simulink model "G474_curLoop_Decouple"  (R2024a)
settings: Solver=FixedStepAuto  StartTime=0.0  StopTime=10  FixedStep=0.0001  RelTol=1e-3  EnableMultiTasking=on
values from neighbouring files (symbols this model uses):
  currentKi = 1.5    [ACM4010.sldd]
  currentKp = 3.5    [ACM4010.sldd]
  flux = 0.006    [ACM4010.sldd]
  J = 6.0E-6    [ACM4010.sldd]
  Ld = 0.0002    [ACM4010.sldd]
  Lq = 0.0002    [ACM4010.sldd]
  Pn = 5.0    [ACM4010.sldd]
undefined symbols (not defined in the file or in its folder): DiscIntNeverNeededParam, sigbuilder_block
libraries: mcbcontrolslib x5, slpidlib x2, mcbplantlib x1, autolibpmsminterior x1
settings Model: DataDictionary=ACM4010.sldd  Creator=zizhong  LastModifiedBy=zizhong
settings OptimizationCC: DefaultParameterBehavior=Inlined  UseDivisionForNetSlopeComputation=on  GainParamInheritBuiltInType=on  UseFloatMulNetSlope=on  InlineInvariantSignals=on  PassReuseOutputArgsAs=Individual arguments  ZeroExternalMemoryAtStartup=off  ZeroInternalMemoryAtStartup=off  NoFixptDivByZeroProtection=on  EfficientFloat2IntCast=on  LifeSpan=1  MaxStackSize=64  OptimizeBlockOrder=speed  DifferentSizesBufferReuse=on  EfficientTunableParamExpr=on
settings DebuggingCC: ParameterTunabilityLossMsg=error
settings HardwareCC: ProdBitPerPointer=32  ProdBitPerSizeT=32  ProdBitPerPtrDiffT=32  ProdLargestAtomicInteger=Long  ProdLargestAtomicFloat=Double  ProdWordSize=32  ProdLongLongMode=on  ProdHWDeviceType=ARM Compatible->ARM Cortex-M
settings SFSimCC: MATLABDynamicMemAlloc=off  SimTargetLang=C++
settings RTWCC: Description=Embedded Coder  SystemTargetFile=ert.tlc  TemplateMakefile=ert_default_tmf  Toolchain=GNU Tools for ARM Embedded Processors
settings CodeAppCC: ForceParamTrailComments=on  IgnoreCustomStorageClasses=off  OperatorAnnotations=on  SimulinkDataObjDesc=on  SFDataObjDesc=on  CustomSymbolStrGlobalVar=rt$N$M  CustomSymbolStrType=$N$M  CustomSymbolStrFcn=$N$M$F  CustomSymbolStrMacro=$N$M  InsertBlockDesc=on
settings ERTTargetCC: TargetLangStandard=C99 (ISO)  CodeReplacementLibrary=ARM Cortex-M  IncludeMdlTerminateFcn=off  CombineSignalStateStructs=on  SupportComplex=off  SupportNonInlinedSFcns=on  ExtModeTransport=3  ExtModeStaticAlloc=on  ExtModeStaticAllocSize=2048  ExtModeMexFile=ext_xcp  ExtModeIntrfLevel=Level2 - Open  InlinedParameterPlacement=NonHierarchical  ERTCustomFileTemplate=example_file_process.tlc  ERTFilePackagingFormat=CompactWithDataFile

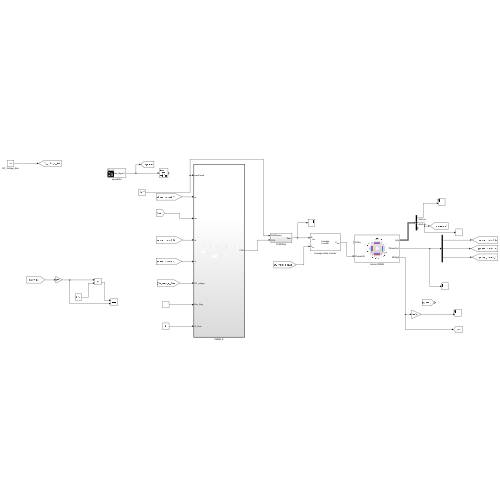
[thumbnail: Simulink's stored preview of the top-level diagram]
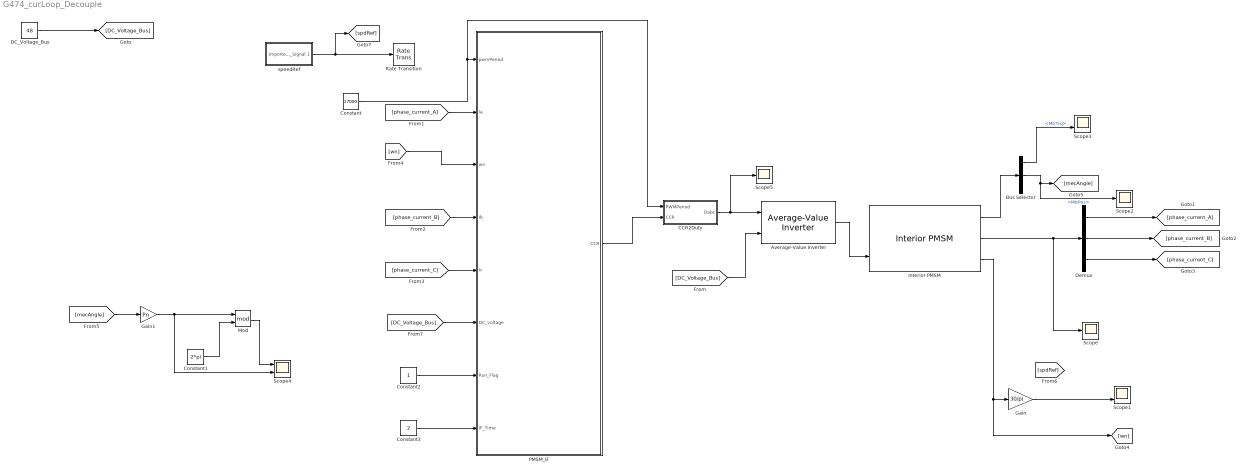
== system G474_curLoop_Decouple ==
  Average-Value Inverter : mcbplantlib/Average-Value Inverter
      settings: LibrarySourceBlock=mcblib/Electrical Systems/Inverters/Average-Value Inverter
  Bus Selector : BusSelector  OutputSignals=MtrTrq,MtrPos,PwrInfo.PwrTrnsfrd
  CCR2Duty : Subsystem
  Constant : Constant  Value=17000
  Constant1 : Constant  Value=2*pi
  Constant2 : Constant
  Constant3 : Constant  Value=2  OutDataTypeStr=single
  DC_Voltage_Bus : Constant  Value=48
  Demux : Demux  Outputs=3
  Gain : Gain  Gain=30/pi
  Gain1 : Gain  Gain=Pn
  Interior PMSM : autolibpmsminterior/Interior PMSM  port_config=Torque  sim_type=Discrete  Ts=0.0001  P=Pn  Rs=Rs  Ldq=[Ld Lq]  KConstText=Permanent flux linkage constant (lambda_pm):  lambda_pm=flux  Ke=159.9771  mechanical=[J,0.924e-4,0]  idq0=[0 0]  theta_init=0  omega_init=0  KConst=flux  lambda_pm_calc=flux  Kt=0.07  RefBlkName='autolibpmsminterior/Interior PMSM'  aMode=5
      settings: LibrarySourceBlock=mcblib/Electrical Systems/Motors/Interior PMSM
  Mod : Math  Operator=mod
  PMSM_IF : Subsystem  TreatAsAtomicUnit=on
      settings: MinAlgLoopOccurrences=on
  Rate Transition : RateTransition
  Scope : Scope
  Scope1 : Scope  NumInputPorts=2
  Scope2 : Scope
  Scope3 : Scope  NumInputPorts=2
  Scope4 : Scope  NumInputPorts=2
  Scope5 : Scope
  speedRef : Subsystem  Tag=STV Subsys  LoadFcn=sigbuilder_block('load');  StartFcn=sigbuilder_block('start');  StopFcn=sigbuilder_block('stop');  ClipboardFcn=sigbuilder_block('clipboard');  mask(Sigbuilder block){tuvar=[0:10]}
      mask help: Simulink:masks:SigbuilderBlock_MD
      mask init:
      | if ~strcmp(get_param(bdroot(gcbh),'SimulationStatus'),'stopped') tuvar = sigbuilder_block('maskInit'); end
      settings: CopyFcn=sigbuilder_block('copy');  DeleteFcn=sigbuilder_block('delete');  ModelCloseFcn=sigbuilder_block('modelClose');  PreSaveFcn=sigbuilder_block('preSave');  PauseFcn=sigbuilder_block('pause');  ContinueFcn=sigbuilder_block('continue');  NameChangeFcn=sigbuilder_block('namechange');  OpenFcn=sigbuilder_block('open',[5.5 36 1269 593 ]);  CloseFcn=sigbuilder_block('close');
      mask Display: plot(0, 0, 100, 100,[2, 2, 32, 32, 2], [68, 8, 8, 68, 68],[32, 2], [38, 38], [32, 19, 2],[53, 60, 44], [32, 17, 17, 2],[16, 16, 31, 31]);txt = getActiveGroup(gcbh);text(2, 100, txt,'verticalAlignment', 'top');
  wires:
  Demux/3 -> [phase_current_C]
  Interior PMSM/2 -> Scope/1, Demux/1
  Average-Value Inverter/1 -> Interior PMSM/2
  CCR2Duty/1(Dabc) -> Scope5/1, Average-Value Inverter/1
  [DC_Voltage_Bus] -> Average-Value Inverter/2
  Bus Selector/1 -> Scope3/2  "<MtrTrq>"
  Gain1/1 -> Scope4/2, Mod/1
  Interior PMSM/3 -> [wn], Gain/1
  Interior PMSM/1 -> Bus Selector/1
  Constant1/1 -> Mod/2
  Demux/1 -> [phase_current_A]
  speedRef/1(Imported_Signal 1) -> Rate Transition/1, [spdRef]
  [mecAngle] -> Gain1/1
  [phase_current_C] -> PMSM_IF/5(Ic)
  Constant/1 -> CCR2Duty/1(PWMPeriod), PMSM_IF/1(pwmPeriod)
  [phase_current_A] -> PMSM_IF/2(Ia)
  Gain/1 -> Scope1/2
  Mod/1 -> Scope4/1
  [phase_current_B] -> PMSM_IF/4(Ib)
  Bus Selector/2 -> Scope2/1, [mecAngle]  "<MtrPos>"
  Demux/2 -> [phase_current_B]
  DC_Voltage_Bus/1 -> [DC_Voltage_Bus]
  [DC_Voltage_Bus] -> PMSM_IF/6(DC_voltage)
  Constant2/1 -> PMSM_IF/7(Run_Flag)
  PMSM_IF/1(CCR) -> CCR2Duty/2(CCR)
  Constant3/1 -> PMSM_IF/8(IF_Time)
  [wn] -> PMSM_IF/3(wn)

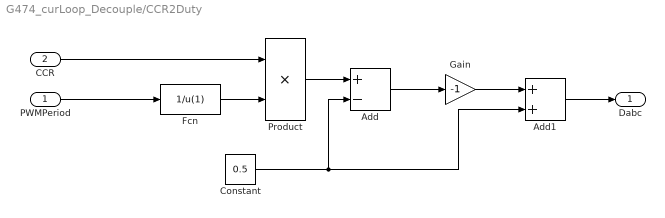
== system G474_curLoop_Decouple/CCR2Duty ==
  PWMPeriod : Inport
  CCR : Inport  Port=2
  Add : Sum  Inputs=+-
  Add1 : Sum
  Constant : Constant  Value=0.5
  Fcn : Fcn  Expr=1/u(1)
  Gain : Gain  Gain=-1
  Product : Product
  Dabc : Outport
  wires:
  PWMPeriod/1 -> Fcn/1
  Fcn/1 -> Product/2
  CCR/1 -> Product/1
  Product/1 -> Add/1
  Constant/1 -> Add1/2, Add/2
  Add/1 -> Gain/1
  Gain/1 -> Add1/1
  Add1/1 -> Dabc/1

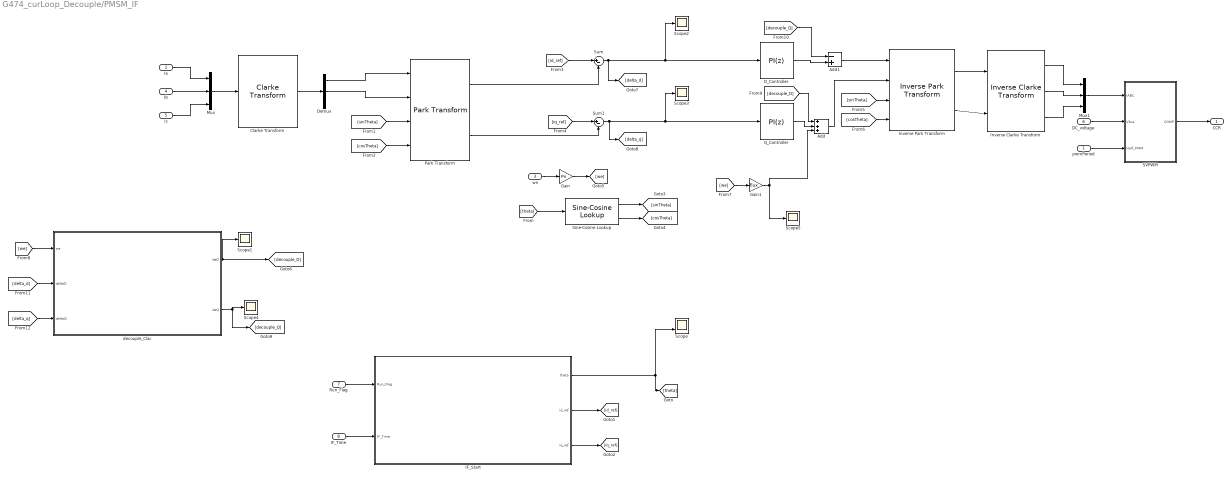
== system G474_curLoop_Decouple/PMSM_IF ==
  pwmPeriod : Inport
  Ia : Inport  Port=2
  wn : Inport  Port=3
  Ib : Inport  Port=4
  Ic : Inport  Port=5
  DC_voltage : Inport  Port=6
  Run_Flag : Inport  Port=7
  IF_Time : Inport  Port=8
  Add : Sum  Inputs=+++
  Add1 : Sum  Inputs=-+
  Clarke Transform : mcbcontrolslib/Clarke Transform  VariantControl=Variant2  PhaseInput=Three inputs  EnPowerInv=off
      settings: LibrarySourceBlock=mcbhdllib/Controls/Math Transforms/Clarke Transform
  D_Controller : slpidlib/PID Controller  Controller=PI  Form=Parallel  TimeDomain=Discrete-time  UseExternalTs=off  SampleTime=-1  IntegratorMethod=Forward Euler  FilterMethod=Forward Euler  ControllerParametersSource=internal  P=currentKp  I=currentKi  UseKiTs=off  D=0  UseExternalDerivativeSource=off  N=100  UseFilter=on  TunerSelectOption=Transfer Function Based (PID Tuner App)  InitialConditionSource=internal  InitialConditionForIntegrator=0  InitialConditionForFilter=0  DifferentiatorICPrevScaledInput=0  ExternalReset=none  TrackingMode=off  Kt=1  LimitOutput=on  SatLimitsSource=internal  UpperSaturationLimit=12  LowerSaturationLimit=-12  LinearizeAsGain=on  AntiWindupMode=clamping  Kb=1  LimitIntegrator=off  UpperIntegratorSaturationLimit=inf  LowerIntegratorSaturationLimit=-inf  PGainOutDataTypeStr=single  PProdOutDataTypeStr=single  POutMin=[]  POutMax=[]  IGainOutDataTypeStr=int16  IProdOutDataTypeStr=int16  IOutMin=[]  IOutMax=[]  DOutMin=[]  DOutMax=[]  NOutMin=[]  NOutMax=[]  SumOutDataTypeStr=single  SumOutMin=[]  SumOutMax=[]  SaturationOutDataTypeStr=single  SaturationOutMin=[]  SaturationOutMax=[]  PParamMin=[]  PParamMax=[]  IParamMin=[]  IParamMax=[]  DParamMin=[]  DParamMax=[]  NParamMin=[]  NParamMax=[]  KbParamMin=[]  KbParamMax=[]  KtParamMin=[]  KtParamMax=[]  KbOutMin=[]  KbOutMax=[]  KtOutMin=[]  KtOutMax=[]  IntegratorOutMin=[]  IntegratorOutMax=[]  FilterOutMin=[]  FilterOutMax=[]  SumI1OutMin=[]  SumI1OutMax=[]  SumI2OutMin=[]  SumI2OutMax=[]  SumI3OutMin=[]  SumI3OutMax=[]  SumI4OutMin=[]  SumI4OutMax=[]  SumDOutMin=[]  SumDOutMax=[]  DifferentiatorOutMin=[]  DifferentiatorOutMax=[]  FilterDiffOutCoefMin=[]  FilterDiffOutCoefMax=[]  ReciprocalOutMin=[]  ReciprocalOutMax=[]  SumDenOutMin=[]  SumDenOutMax=[]  SumNumOutMin=[]  SumNumOutMax=[]  DivideOutMin=[]  DivideOutMax=[]  UdiffTsProdOutMin=[]  UdiffTsProdOutMax=[]  NTsProdOutMin=[]  NTsProdOutMax=[]  UintegralTsProdOutMin=[]  UintegralTsProdOutMax=[]  UngainTsProdOutMin=[]  UngainTsProdOutMax=[]  ClampingZeroOutDataTypeStr=Inherit: Inherit via back propagation  ClampingZeroOutMin=[]  ClampingZeroOutMax=[]  FilterDenConstantOutDataTypeStr=Inherit: Inherit via back propagation  FilterDenConstantOutMin=[]  FilterDenConstantOutMax=[]  PCopyOutDataTypeStr=Inherit: Inherit via back propagation  PCopyOutMin=[]  PCopyOutMax=[]  NCopyOutDataTypeStr=Inherit: Inherit via back propagation  NCopyOutMin=[]  NCopyOutMax=[]  IntegratorContinuousStateAttributes=''  IntegratorStateMustResolveToSignalObject=off  IntegratorRTWStateStorageClass=Auto  FilterContinuousStateAttributes=''  FilterStateMustResolveToSignalObject=off  FilterRTWStateStorageClass=Auto  ParallelPVariant=InternalParameters  IdealPVariant=Disabled  IVariant=InternalParameters  DVariant=Disabled  IntegratorVariant=Discrete  SatVariant=Enabled  AWVariant=DiscClampingParallel  PCopyVariant=Disabled  TRVariant=Disabled  FdbkBlocksVariant=Forward  IdealPFdbkVariant=Disabled  SatFdbkVariant=Disabled  DerivativeFilterVariant=Disabled  NVariant=Disabled  NCopyVariant=Disabled_SignalSpec  FilterICVariant=Disabled  IntegratorICVariant=InternalICs  ExternalResetVariant=Disabled  TRSumVariant=Passthrough  SumFdbkVariant=Disabled  SumVariant=Sum_PI  TsampFilterVariant=InternalTs  TsampNgainVariant=Passthrough  TsampIntegralVariant=Disabled_SignalSpec  ExternalSaturationOutDataTypeStr=Inherit: Same as second input  DerivativeSourceVariant=Disabled
  Demux : Demux  Outputs=3
  Gain : Gain  Gain=Pn
  Gain1 : Gain  Gain=flux
  IF_Start : Subsystem  TreatAsAtomicUnit=on
      settings: MinAlgLoopOccurrences=on
  Inverse Clarke Transform : mcbcontrolslib/Inverse Clarke Transform  PhaseInput=Two inputs  EnPowerInv=off
      settings: LibrarySourceBlock=mcbhdllib/Controls/Math Transforms/Inverse Clarke Transform
  Inverse Park Transform : mcbcontrolslib/Inverse Park Transform  PhaseInput=Two inputs  AxisAlignment=D-axis  ThetaInput=Sine and Cosine electrical position  AngleInput=Per-unit  N_points=1024
      settings: LibrarySourceBlock=mcbhdllib/Controls/Math Transforms/Inverse Park Transform
  Mux : Mux  Inputs=3
  Mux1 : Mux  Inputs=3
  Park Transform : mcbcontrolslib/Park Transform  PhaseInput=Two inputs  AxisAlignment=D-axis  ThetaInput=Sine and Cosine electrical position  AngleInput=Per-unit  N_points=1024
      settings: LibrarySourceBlock=mcbhdllib/Controls/Math Transforms/Park Transform
  Q_Controller : slpidlib/PID Controller  Controller=PI  Form=Parallel  TimeDomain=Discrete-time  UseExternalTs=off  SampleTime=-1  IntegratorMethod=Forward Euler  FilterMethod=Forward Euler  ControllerParametersSource=internal  P=currentKp  I=currentKi  UseKiTs=off  D=0  UseExternalDerivativeSource=off  N=100  UseFilter=on  TunerSelectOption=Transfer Function Based (PID Tuner App)  InitialConditionSource=internal  InitialConditionForIntegrator=0  InitialConditionForFilter=0  DifferentiatorICPrevScaledInput=0  ExternalReset=none  TrackingMode=off  Kt=1  LimitOutput=on  SatLimitsSource=internal  UpperSaturationLimit=12  LowerSaturationLimit=-12  LinearizeAsGain=on  AntiWindupMode=clamping  Kb=1  LimitIntegrator=off  UpperIntegratorSaturationLimit=inf  LowerIntegratorSaturationLimit=-inf  PGainOutDataTypeStr=single  PProdOutDataTypeStr=single  POutMin=[]  POutMax=[]  IGainOutDataTypeStr=int16  IProdOutDataTypeStr=int16  IOutMin=[]  IOutMax=[]  DOutMin=[]  DOutMax=[]  NOutMin=[]  NOutMax=[]  SumOutDataTypeStr=single  SumOutMin=[]  SumOutMax=[]  SaturationOutDataTypeStr=single  SaturationOutMin=[]  SaturationOutMax=[]  PParamMin=[]  PParamMax=[]  IParamMin=[]  IParamMax=[]  DParamMin=[]  DParamMax=[]  NParamMin=[]  NParamMax=[]  KbParamMin=[]  KbParamMax=[]  KtParamMin=[]  KtParamMax=[]  KbOutMin=[]  KbOutMax=[]  KtOutMin=[]  KtOutMax=[]  IntegratorOutMin=[]  IntegratorOutMax=[]  FilterOutMin=[]  FilterOutMax=[]  SumI1OutMin=[]  SumI1OutMax=[]  SumI2OutMin=[]  SumI2OutMax=[]  SumI3OutMin=[]  SumI3OutMax=[]  SumI4OutMin=[]  SumI4OutMax=[]  SumDOutMin=[]  SumDOutMax=[]  DifferentiatorOutMin=[]  DifferentiatorOutMax=[]  FilterDiffOutCoefMin=[]  FilterDiffOutCoefMax=[]  ReciprocalOutMin=[]  ReciprocalOutMax=[]  SumDenOutMin=[]  SumDenOutMax=[]  SumNumOutMin=[]  SumNumOutMax=[]  DivideOutMin=[]  DivideOutMax=[]  UdiffTsProdOutMin=[]  UdiffTsProdOutMax=[]  NTsProdOutMin=[]  NTsProdOutMax=[]  UintegralTsProdOutMin=[]  UintegralTsProdOutMax=[]  UngainTsProdOutMin=[]  UngainTsProdOutMax=[]  ClampingZeroOutDataTypeStr=Inherit: Inherit via back propagation  ClampingZeroOutMin=[]  ClampingZeroOutMax=[]  FilterDenConstantOutDataTypeStr=Inherit: Inherit via back propagation  FilterDenConstantOutMin=[]  FilterDenConstantOutMax=[]  PCopyOutDataTypeStr=Inherit: Inherit via back propagation  PCopyOutMin=[]  PCopyOutMax=[]  NCopyOutDataTypeStr=Inherit: Inherit via back propagation  NCopyOutMin=[]  NCopyOutMax=[]  IntegratorContinuousStateAttributes=''  IntegratorStateMustResolveToSignalObject=off  IntegratorRTWStateStorageClass=Auto  FilterContinuousStateAttributes=''  FilterStateMustResolveToSignalObject=off  FilterRTWStateStorageClass=Auto  ParallelPVariant=InternalParameters  IdealPVariant=Disabled  IVariant=InternalParameters  DVariant=Disabled  IntegratorVariant=Discrete  SatVariant=Enabled  AWVariant=DiscClampingParallel  PCopyVariant=Disabled  TRVariant=Disabled  FdbkBlocksVariant=Forward  IdealPFdbkVariant=Disabled  SatFdbkVariant=Disabled  DerivativeFilterVariant=Disabled  NVariant=Disabled  NCopyVariant=Disabled_SignalSpec  FilterICVariant=Disabled  IntegratorICVariant=InternalICs  ExternalResetVariant=Disabled  TRSumVariant=Passthrough  SumFdbkVariant=Disabled  SumVariant=Sum_PI  TsampFilterVariant=InternalTs  TsampNgainVariant=Passthrough  TsampIntegralVariant=Disabled_SignalSpec  ExternalSaturationOutDataTypeStr=Inherit: Same as second input  DerivativeSourceVariant=Disabled
  SVPWM : Subsystem  TreatAsAtomicUnit=on
      settings: MinAlgLoopOccurrences=on
  Scope : Scope  NumInputPorts=2
  Scope{1..5} (5 alike) : Scope
  Sine-Cosine Lookup : mcbcontrolslib/Sine-Cosine Lookup  AngleInput=Radians  N_points=1024  DatatypeInput=Inherit from input  Datatype=single
      settings: LibrarySourceBlock=mcblib/Controls/Math Transforms/Sine-Cosine Lookup
  Sum : Sum  Inputs=|+-
  Sum1 : Sum  Inputs=|+-
  decouple_Clac : Subsystem
  CCR : Outport
  wires:
  [theta] -> Sine-Cosine Lookup/1
  Mux/1 -> Clarke Transform/1
  Ia/1 -> Mux/1
  Ib/1 -> Mux/2
  Ic/1 -> Mux/3
  Sine-Cosine Lookup/1 -> [sinTheta]
  Sine-Cosine Lookup/2 -> [cosTheta]
  [sinTheta] -> Park Transform/3
  [cosTheta] -> Park Transform/4
  Clarke Transform/1 -> Demux/1
  Demux/2 -> Park Transform/2
  Demux/1 -> Park Transform/1
  Park Transform/1 -> Sum/2
  Park Transform/2 -> Sum1/2
  [id_ref] -> Sum/1
  [iq_ref] -> Sum1/1
  [sinTheta] -> Inverse Park Transform/3
  [cosTheta] -> Inverse Park Transform/4
  Inverse Park Transform/1 -> Inverse Clarke Transform/1
  Inverse Park Transform/2 -> Inverse Clarke Transform/2
  Inverse Clarke Transform/1 -> Mux1/1
  Inverse Clarke Transform/2 -> Mux1/2
  Inverse Clarke Transform/3 -> Mux1/3
  Mux1/1 -> SVPWM/1(IABC)
  DC_voltage/1 -> SVPWM/2(Vbus)
  pwmPeriod/1 -> SVPWM/3(Half_PWM)
  SVPWM/1(COMP) -> CCR/1
  IF_Start/1(theta) -> Scope/2, [theta]
  Run_Flag/1 -> IF_Start/1(Run_Flag)
  IF_Time/1 -> IF_Start/2(IF_Time)
  IF_Start/2(id_ref) -> [id_ref]
  IF_Start/3(iq_ref) -> [iq_ref]
  Add/1 -> Inverse Park Transform/2
  Add1/1 -> Inverse Park Transform/1
  D_Controller/1 -> Add1/2
  wn/1 -> Gain/1
  Gain/1 -> [we]
  [we] -> Gain1/1
  Q_Controller/1 -> Add/2
  [decouple_D] -> Add/1
  [decouple_Q] -> Add1/1
  Gain1/1 -> Add/3, Scope5/1
  decouple_Clac/2(deQ) -> [decouple_Q], Scope4/1
  decouple_Clac/1(deD) -> [decouple_D], Scope1/1
  [we] -> decouple_Clac/1(we)
  [delta_d] -> decouple_Clac/2(deltaD)
  [delta_q] -> decouple_Clac/3(deltaQ)
  Sum1/1 -> [delta_q], Q_Controller/1, Scope3/1
  Sum/1 -> [delta_d], D_Controller/1, Scope2/1

== system G474_curLoop_Decouple/speedRef ==
  Demux : Demux  Tag=STV Demux  Outputs=1
      settings: DisplayOption=none
  FromWs : FromWorkspace  Tag=STV FromWs  VariableName=tuvar
      SigBuilderData=|
      | common.afterFinalStr = 'Extrapolate'
      | common.sampleTime = 0
      | dataSet.timeRange = [0 10]
      | dataSet.name = 'Sheet1'
      | sbobj.Groups.Name = 'Sheet1'
      | sbobj.Groups.Signals.Name = 'Imported_Signal 1'
      | sbobj.Groups.Signals.XData = [0 1 2 3 4 5 5.96 7 8 9 10]
      | sbobj.Groups.Signals.YData = [3580 3680 3785 3660 3855 3595 3670 3535 2755 3650 3760]
  Imported_Signal 1 : Outport  Tag=STV Outport
  wires:
  Demux/1 -> Imported_Signal 1/1
  FromWs/1 -> Demux/1

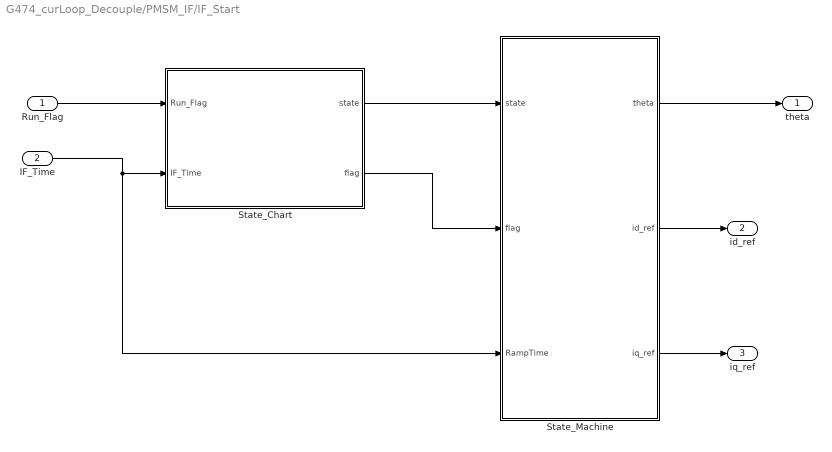
== system G474_curLoop_Decouple/PMSM_IF/IF_Start ==
  Run_Flag : Inport
  IF_Time : Inport  Port=2
  State_Chart : Stateflow chart
      settings: MinAlgLoopOccurrences=on
  State_Machine : Subsystem  TreatAsAtomicUnit=on
      settings: MinAlgLoopOccurrences=on
  theta : Outport
  id_ref : Outport  Port=2
  iq_ref : Outport  Port=3
  wires:
  State_Machine/3(iq_ref) -> iq_ref/1
  State_Chart/2(flag) -> State_Machine/2(flag)
  IF_Time/1 -> State_Machine/3(RampTime), State_Chart/2(IF_Time)
  State_Chart/1(state) -> State_Machine/1(state)
  State_Machine/1(theta) -> theta/1
  State_Machine/2(id_ref) -> id_ref/1
  Run_Flag/1 -> State_Chart/1(Run_Flag)

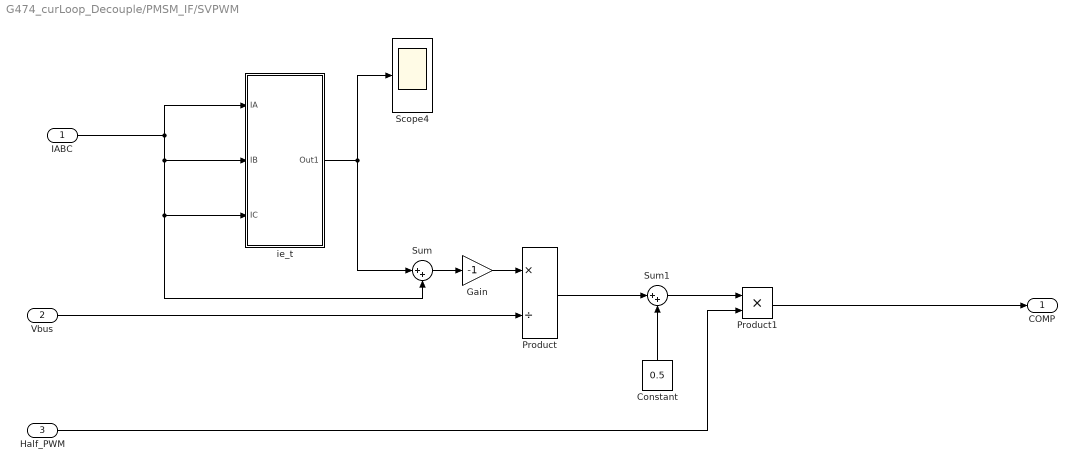
== system G474_curLoop_Decouple/PMSM_IF/SVPWM ==
  IABC : Inport
  Vbus : Inport  Port=2
  Half_PWM : Inport  Port=3
  Constant : Constant  Value=0.5
  Gain : Gain  Gain=-1
  Product : Product  Inputs=*/
  Product1 : Product
  Scope4 : Scope
  Sum : Sum  Inputs=|++
  Sum1 : Sum  Inputs=|++
  ie_t : Subsystem
  COMP : Outport
  wires:
  IABC/1 -> ie_t/3(IC), Sum/2, ie_t/2(IB), ie_t/1(IA)
  Half_PWM/1 -> Product1/2
  Gain/1 -> Product/1
  ie_t/1(Out1) -> Sum/1, Scope4/1
  Sum/1 -> Gain/1
  Sum1/1 -> Product1/1
  Constant/1 -> Sum1/2
  Product/1 -> Sum1/1
  Vbus/1 -> Product/2
  Product1/1 -> COMP/1

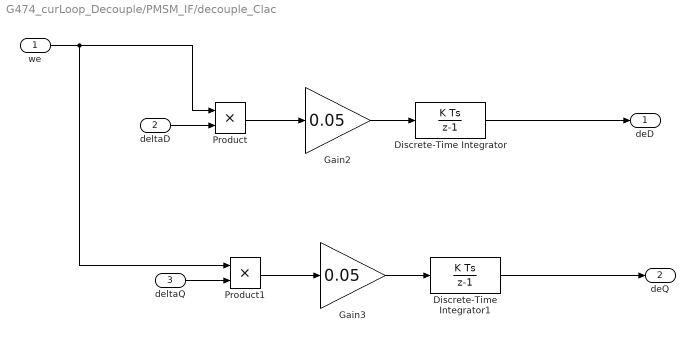
== system G474_curLoop_Decouple/PMSM_IF/decouple_Clac ==
  we : Inport
  deltaD : Inport  Port=2
  deltaQ : Inport  Port=3
  Discrete-Time Integrator : DiscreteIntegrator  SampleTime=-1  LimitOutput=on  UpperSaturationLimit=8  LowerSaturationLimit=-8  ICPrevOutput=DiscIntNeverNeededParam  ICPrevScaledInput=DiscIntNeverNeededParam
  Discrete-Time Integrator1 : DiscreteIntegrator  SampleTime=-1  LimitOutput=on  UpperSaturationLimit=8  LowerSaturationLimit=-8  ICPrevOutput=DiscIntNeverNeededParam  ICPrevScaledInput=DiscIntNeverNeededParam
  Gain2 : Gain  Gain=0.05
  Gain3 : Gain  Gain=0.05
  Product : Product
  Product1 : Product
  deD : Outport
  deQ : Outport  Port=2
  wires:
  Gain2/1 -> Discrete-Time Integrator/1
  Product/1 -> Gain2/1
  we/1 -> Product1/1, Product/1
  Product1/1 -> Gain3/1
  Gain3/1 -> Discrete-Time Integrator1/1
  Discrete-Time Integrator/1 -> deD/1
  deltaQ/1 -> Product1/2
  deltaD/1 -> Product/2
  Discrete-Time Integrator1/1 -> deQ/1

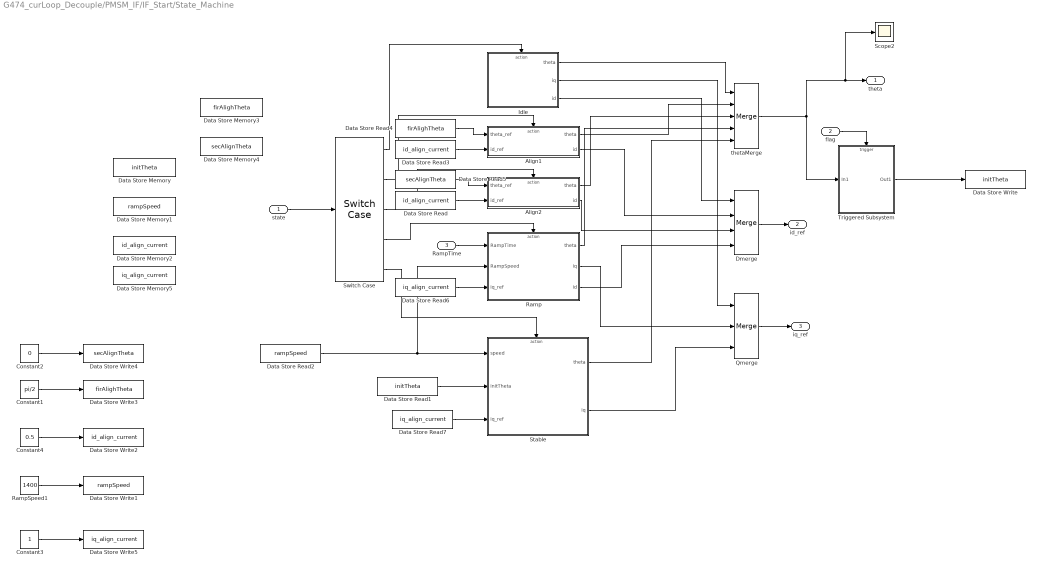
== system G474_curLoop_Decouple/PMSM_IF/IF_Start/State_Machine ==
  state : Inport
  flag : Inport  Port=2
  RampTime : Inport  Port=3
  Align1 : Subsystem  TreatAsAtomicUnit=on
  Align2 : Subsystem  TreatAsAtomicUnit=on
  Constant1 : Constant  Value=pi/2  OutDataTypeStr=single
  Constant2 : Constant  Value=0  OutDataTypeStr=single
  Constant3 : Constant  OutDataTypeStr=single
  Constant4 : Constant  Value=0.5  OutDataTypeStr=single
  Data Store Memory : DataStoreMemory  DataStoreName=initTheta  WriteAfterWriteMsg=warning  ShowAdditionalParam=off
  Data Store Memory1 : DataStoreMemory  DataStoreName=rampSpeed  WriteAfterWriteMsg=warning  ShowAdditionalParam=off
  Data Store Memory2 : DataStoreMemory  DataStoreName=id_align_current  WriteAfterWriteMsg=warning  ShowAdditionalParam=off
  Data Store Memory3 : DataStoreMemory  DataStoreName=firAlighTheta  WriteAfterWriteMsg=warning  ShowAdditionalParam=off
  Data Store Memory4 : DataStoreMemory  DataStoreName=secAlignTheta  WriteAfterWriteMsg=warning  ShowAdditionalParam=off
  Data Store Memory5 : DataStoreMemory  DataStoreName=iq_align_current  WriteAfterWriteMsg=warning  ShowAdditionalParam=off
  Data Store Read : DataStoreRead  DataStoreName=id_align_current  IndexOptions=Index vector (dialog)  Indices=1  OutputSizes=1
  Data Store Read1 : DataStoreRead  DataStoreName=initTheta  IndexOptions=Index vector (dialog)  Indices=1  OutputSizes=1
  Data Store Read2 : DataStoreRead  DataStoreName=rampSpeed  IndexOptions=Index vector (dialog)  Indices=1  OutputSizes=1
  Data Store Read3 : DataStoreRead  DataStoreName=id_align_current  IndexOptions=Index vector (dialog)  Indices=1  OutputSizes=1
  Data Store Read4 : DataStoreRead  DataStoreName=firAlighTheta  IndexOptions=Index vector (dialog)  Indices=1  OutputSizes=1
  Data Store Read5 : DataStoreRead  DataStoreName=secAlignTheta  IndexOptions=Index vector (dialog)  Indices=1  OutputSizes=1
  Data Store Read6 : DataStoreRead  DataStoreName=iq_align_current  IndexOptions=Index vector (dialog)  Indices=1  OutputSizes=1
  Data Store Read7 : DataStoreRead  DataStoreName=iq_align_current  IndexOptions=Index vector (dialog)  Indices=1  OutputSizes=1
  Data Store Write : DataStoreWrite  DataStoreName=initTheta  IndexOptions=Index vector (dialog)  Indices=1  OutputSizes=1
  Data Store Write1 : DataStoreWrite  DataStoreName=rampSpeed  IndexOptions=Index vector (dialog)  Indices=1  OutputSizes=1
  Data Store Write2 : DataStoreWrite  DataStoreName=id_align_current  IndexOptions=Index vector (dialog)  Indices=1  OutputSizes=1
  Data Store Write3 : DataStoreWrite  DataStoreName=firAlighTheta  IndexOptions=Index vector (dialog)  Indices=1  OutputSizes=1
  Data Store Write4 : DataStoreWrite  DataStoreName=secAlignTheta  IndexOptions=Index vector (dialog)  Indices=1  OutputSizes=1
  Data Store Write5 : DataStoreWrite  DataStoreName=iq_align_current  IndexOptions=Index vector (dialog)  Indices=1  OutputSizes=1
  Dmerge : Merge  Inputs=4
  Idle : Subsystem  TreatAsAtomicUnit=on
  Qmerge : Merge  Inputs=3
  Ramp : Subsystem  TreatAsAtomicUnit=on
  RampSpeed1 : Constant  Value=1400  OutDataTypeStr=single
  Scope2 : Scope
  Stable : Subsystem  TreatAsAtomicUnit=on
  Switch Case : SwitchCase  CaseConditions={0, 1, 2, 3, 4}  ShowDefaultCase=off
  Triggered Subsystem : Subsystem  TreatAsAtomicUnit=on
  thetaMerge : Merge  Inputs=5
  theta : Outport
  id_ref : Outport  Port=2
  iq_ref : Outport  Port=3
  wires:
  Align1/2(id) -> Dmerge/2
  Data Store Read4/1 -> Align1/1(theta_ref)
  Switch Case/5 -> Stable/Action
  Switch Case/1 -> Idle/Action
  Data Store Read/1 -> Align2/2(id_ref)
  Stable/2(iq) -> Qmerge/3
  Ramp/2(iq) -> Qmerge/2
  Switch Case/2 -> Align1/Action
  Data Store Read2/1 -> Ramp/2(RampSpeed), Stable/1(speed)
  Data Store Read7/1 -> Stable/3(iq_ref)
  Data Store Read5/1 -> Align2/1(theta_ref)
  Data Store Read6/1 -> Ramp/3(iq_ref)
  Ramp/3(id) -> Dmerge/4
  Align1/1(theta) -> thetaMerge/2
  Dmerge/1 -> id_ref/1
  Idle/3(id) -> Dmerge/1
  Ramp/1(theta) -> thetaMerge/4
  Switch Case/3 -> Align2/Action
  Data Store Read3/1 -> Align1/2(id_ref)
  Align2/2(id) -> Dmerge/3
  Idle/2(iq) -> Qmerge/1
  Switch Case/4 -> Ramp/Action
  Align2/1(theta) -> thetaMerge/3
  Idle/1(theta) -> thetaMerge/1
  RampTime/1 -> Ramp/1(RampTime)
  state/1 -> Switch Case/1
  Qmerge/1 -> iq_ref/1
  thetaMerge/1 -> Triggered Subsystem/1(In1), Scope2/1, theta/1
  Stable/1(theta) -> thetaMerge/5
  flag/1 -> Triggered Subsystem/Trigger
  Data Store Read1/1 -> Stable/2(initTheta)
  Triggered Subsystem/1(Out1) -> Data Store Write/1
  RampSpeed1/1 -> Data Store Write1/1
  Constant4/1 -> Data Store Write2/1
  Constant1/1 -> Data Store Write3/1
  Constant2/1 -> Data Store Write4/1
  Constant3/1 -> Data Store Write5/1

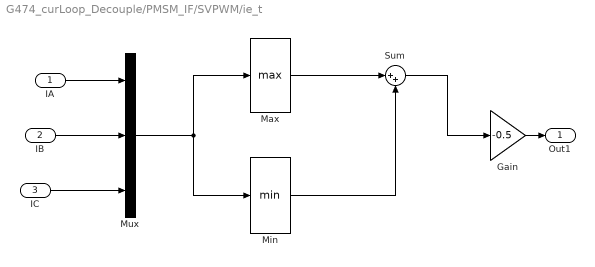
== system G474_curLoop_Decouple/PMSM_IF/SVPWM/ie_t ==
  IA : Inport
  IB : Inport  Port=2
  IC : Inport  Port=3
  Gain : Gain  Gain=-0.5
  Max : MinMax  Function=max
  Min : MinMax
  Mux : Mux  Inputs=3
  Sum : Sum  Inputs=|++
  Out1 : Outport
  wires:
  Max/1 -> Sum/1
  IC/1 -> Mux/3
  Mux/1 -> Min/1, Max/1
  Sum/1 -> Gain/1
  Min/1 -> Sum/2
  IA/1 -> Mux/1
  Gain/1 -> Out1/1
  IB/1 -> Mux/2

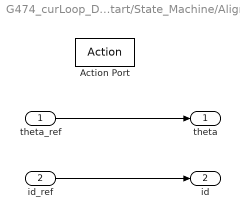
== system G474_curLoop_Decouple/PMSM_IF/IF_Start/State_Machine/Align1 ==
  theta_ref : Inport
  id_ref : Inport  Port=2
  Action Port : ActionPort  ActionPortLabel=case [ 1 ]:
  theta : Outport
  id : Outport  Port=2
  wires:
  theta_ref/1 -> theta/1
  id_ref/1 -> id/1

== system G474_curLoop_Decouple/PMSM_IF/IF_Start/State_Machine/Align2 ==
  theta_ref : Inport
  id_ref : Inport  Port=2
  Action Port : ActionPort  ActionPortLabel=case [ 2 ]:
  theta : Outport
  id : Outport  Port=2
  wires:
  id_ref/1 -> id/1
  theta_ref/1 -> theta/1

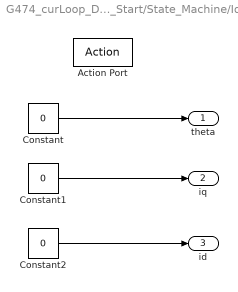
== system G474_curLoop_Decouple/PMSM_IF/IF_Start/State_Machine/Idle ==
  Action Port : ActionPort  ActionPortLabel=case [ 0 ]:
  Constant : Constant  Value=0  OutDataTypeStr=single
  Constant1 : Constant  Value=0  OutDataTypeStr=single
  Constant2 : Constant  Value=0  OutDataTypeStr=single
  theta : Outport
  iq : Outport  Port=2
  id : Outport  Port=3
  wires:
  Constant1/1 -> iq/1
  Constant/1 -> theta/1
  Constant2/1 -> id/1

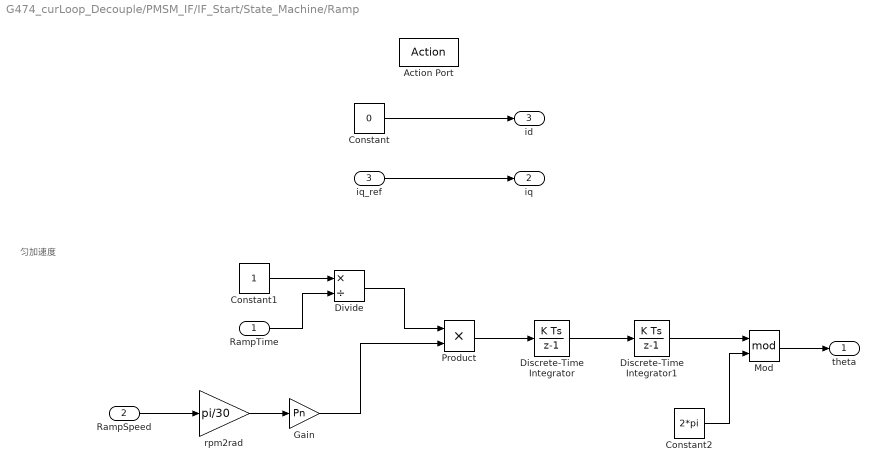
== system G474_curLoop_Decouple/PMSM_IF/IF_Start/State_Machine/Ramp ==
  note: 匀加速度
  RampTime : Inport
  RampSpeed : Inport  Port=2
  iq_ref : Inport  Port=3
  Action Port : ActionPort  ActionPortLabel=case [ 3 ]:
  Constant : Constant  Value=0  OutDataTypeStr=single
  Constant1 : Constant  OutDataTypeStr=single
  Constant2 : Constant  Value=2*pi  OutDataTypeStr=single
  Discrete-Time Integrator : DiscreteIntegrator  SampleTime=-1  ICPrevOutput=DiscIntNeverNeededParam  ICPrevScaledInput=DiscIntNeverNeededParam
  Discrete-Time Integrator1 : DiscreteIntegrator  SampleTime=-1  ICPrevOutput=DiscIntNeverNeededParam  ICPrevScaledInput=DiscIntNeverNeededParam
  Divide : Product  Inputs=*/
  Gain : Gain  Gain=Pn
  Mod : Math  Operator=mod
  Product : Product
  rpm2rad : Gain  Gain=pi/30
  theta : Outport
  iq : Outport  Port=2
  id : Outport  Port=3
  wires:
  Constant/1 -> id/1
  iq_ref/1 -> iq/1
  RampSpeed/1 -> rpm2rad/1
  Constant1/1 -> Divide/1
  RampTime/1 -> Divide/2
  Divide/1 -> Product/1
  rpm2rad/1 -> Gain/1
  Product/1 -> Discrete-Time Integrator/1
  Discrete-Time Integrator/1 -> Discrete-Time Integrator1/1
  Mod/1 -> theta/1
  Constant2/1 -> Mod/2
  Gain/1 -> Product/2
  Discrete-Time Integrator1/1 -> Mod/1

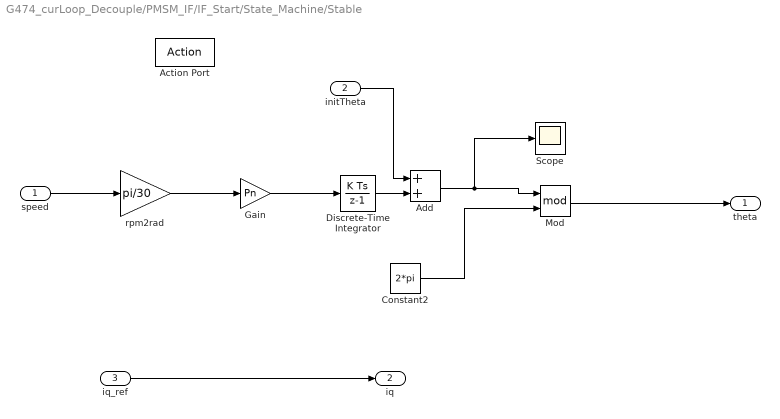
== system G474_curLoop_Decouple/PMSM_IF/IF_Start/State_Machine/Stable ==
  speed : Inport
  initTheta : Inport  Port=2
  iq_ref : Inport  Port=3
  Action Port : ActionPort  ActionPortLabel=case [ 4 ]:
  Add : Sum
  Constant2 : Constant  Value=2*pi  OutDataTypeStr=single
  Discrete-Time Integrator : DiscreteIntegrator  SampleTime=-1  ICPrevOutput=DiscIntNeverNeededParam  ICPrevScaledInput=DiscIntNeverNeededParam
  Gain : Gain  Gain=Pn
  Mod : Math  Operator=mod
  Scope : Scope
  rpm2rad : Gain  Gain=pi/30
  theta : Outport
  iq : Outport  Port=2
  wires:
  rpm2rad/1 -> Gain/1
  speed/1 -> rpm2rad/1
  Gain/1 -> Discrete-Time Integrator/1
  Constant2/1 -> Mod/2
  iq_ref/1 -> iq/1
  Mod/1 -> theta/1
  Discrete-Time Integrator/1 -> Add/2
  Add/1 -> Scope/1, Mod/1
  initTheta/1 -> Add/1

== system G474_curLoop_Decouple/PMSM_IF/IF_Start/State_Machine/Triggered Subsystem ==
  In1 : Inport
  Trigger : TriggerPort  VariantControl=(inherit)
  Out1 : Outport
  wires:
  In1/1 -> Out1/1

== stateflow chart G474_curLoop_Decouple/PMSM_IF/IF_Start/State_Chart ==
  state Ramp
    en:
    state = 3;
  state Idle
    en:
    state = 0;
  state First_Align
    en:
    state = 1;
  state Last_Align
    en:
    state = 2;
  state Stablize
    en:
    state = 4;
  Ramp -> (junction 87) [order 3] : [after(IF_Time * 9999,tick)]{flag = 1}
  (default) -> Idle
  Idle -> First_Align : [Run_Flag == 1]
  First_Align -> Last_Align [order 1] : [after(1000,tick)]
  Last_Align -> Ramp [order 1] : [after(1000,tick)]
  Ramp -> Stablize [order 1] : [after(IF_Time * 10000,tick)]
  First_Align -> Idle [order 2] : [Run_Flag == 0]
  Last_Align -> Idle [order 2] : [Run_Flag == 0]
  Ramp -> Idle [order 2] : [Run_Flag == 0]
  Stablize -> Idle : [Run_Flag == 0]
  data: Run_Flag input; state output; IF_Time input; flag output
